simulink model "pBrake"  (R2024b)
settings: Solver=FixedStepDiscrete  StartTime=0.0  StopTime=1  FixedStep=0.001  RelTol=1e-3  EnableMultiTasking=on
undefined symbols (not defined in the file): pBrakeGain
settings Model: DataDictionary=Master_Dictionary.sldd  EnableAccessToBaseWorkspace=off  Creator=rubyg  LastModifiedBy=oxbro
settings SolverCC: AlgebraicLoopSolver=TrustRegion
settings DataIOCC: ReturnWorkspaceOutputs=off
settings OptimizationCC: DefaultParameterBehavior=Inlined  EnhancedBackFolding=on  PassReuseOutputArgsAs=Individual arguments  ZeroExternalMemoryAtStartup=off  ZeroInternalMemoryAtStartup=off  MaxStackSize=512  OptimizeBlockOrder=speed  DifferentSizesBufferReuse=on  OptimizationCustomize=off  EfficientTunableParamExpr=on
settings DebuggingCC: ParameterTunabilityLossMsg=error  UnconnectedInputMsg=warning  UnconnectedOutputMsg=warning  UnconnectedLineMsg=warning  ArithmeticOperatorsInVariantConditions=warning
settings HardwareCC: ProdBitPerPointer=32  ProdBitPerSizeT=32  ProdBitPerPtrDiffT=32  ProdLargestAtomicInteger=Long  ProdLargestAtomicFloat=Double  ProdWordSize=32  ProdLongLongMode=on  ProdHWDeviceType=ARM Compatible->ARM Cortex-M
settings ModelReferenceCC: EnableRefExpFcnMdlSchedulingChecks=on
settings SFSimCC: MATLABDynamicMemAlloc=off  CustomCodeUndefinedFunction=UseInterfaceOnly
settings RTWCC: Description=Embedded Coder  SystemTargetFile=ert.tlc  HardwareBoard=STM32H7xx Based (Single-core)  TemplateMakefile=ert_default_tmf  CustomHeaderCode="#include \"stm32h7xx_ll_tim.h\""  CustomInitializer=LL_TIM_EnableCounter(TIM2);  Toolchain=GNU Tools for ARM Embedded Processors  GPUComputeCapability=3.5
settings CodeAppCC: ForceParamTrailComments=on  IgnoreCustomStorageClasses=off  OperatorAnnotations=on  SimulinkDataObjDesc=on  SFDataObjDesc=on  InsertBlockDesc=on
settings ERTTargetCC: TargetLangStandard=C99 (ISO)  CodeReplacementLibrary=ARM Cortex-M  ExtModeTransport=3  ExtModeStaticAlloc=on  ExtModeStaticAllocSize=2048  ExtModeMexFile=ext_xcp  ExtModeIntrfLevel=Level2 - Open

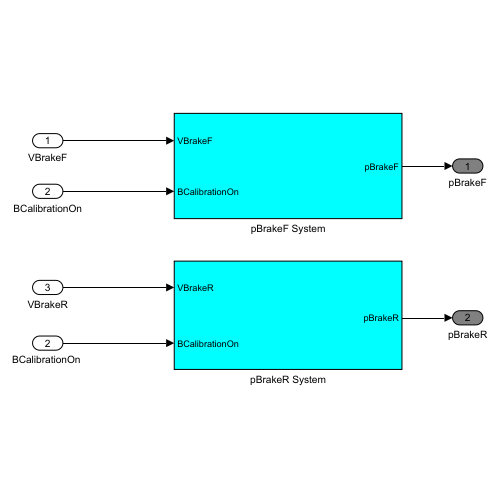
[thumbnail: Simulink's stored preview of the top-level diagram]
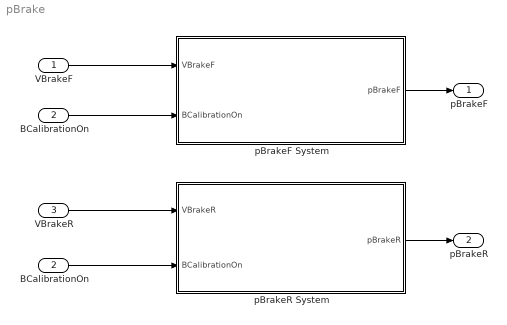
== system pBrake ==
  VBrakeF : Inport
  BCalibrationOn : Inport  Port=2  OutDataTypeStr=boolean
  VBrakeR : Inport  Port=3
  "BCalibrationOn " : InportShadow  Port=2  OutDataTypeStr=boolean
  pBrakeF System : Subsystem
  pBrakeR System : Subsystem
  pBrakeF : Outport  OutDataTypeStr=double  VectorParamsAs1DForOutWhenUnconnected=off
  pBrakeR : Outport  Port=2  OutDataTypeStr=double  VectorParamsAs1DForOutWhenUnconnected=off
  wires:
  BCalibrationOn/1 -> pBrakeF System/2(BCalibrationOn)
  VBrakeF/1 -> pBrakeF System/1(VBrakeF)
  "BCalibrationOn "/1 -> pBrakeR System/2(BCalibrationOn)
  VBrakeR/1 -> pBrakeR System/1(VBrakeR)
  pBrakeF System/1(pBrakeF) -> pBrakeF/1
  pBrakeR System/1(pBrakeR) -> pBrakeR/1

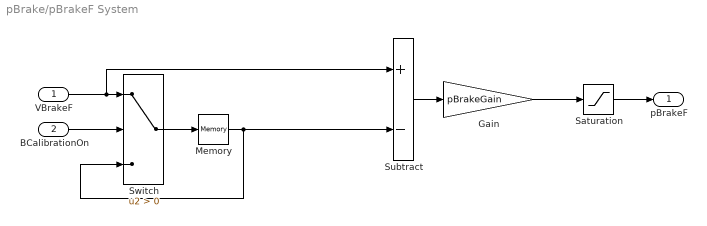
== system pBrake/pBrakeF System ==
  VBrakeF : Inport
  BCalibrationOn : Inport  Port=2  OutDataTypeStr=boolean
  Gain : Gain  Gain=pBrakeGain
  Memory : Memory  InitialCondition=500  InheritSampleTime=on
  Saturation : Saturate  UpperLimit=240  LowerLimit=-80
  Subtract : Sum  Inputs=+-
  Switch : Switch  Criteria=u2 > Threshold  SaturateOnIntegerOverflow=off  InputSameDT=off
  pBrakeF : Outport  VectorParamsAs1DForOutWhenUnconnected=off
  wires:
  VBrakeF/1 -> Subtract/1, Switch/1
  BCalibrationOn/1 -> Switch/2
  Switch/1 -> Memory/1
  Memory/1 -> Switch/3, Subtract/2
  Subtract/1 -> Gain/1
  Saturation/1 -> pBrakeF/1
  Gain/1 -> Saturation/1

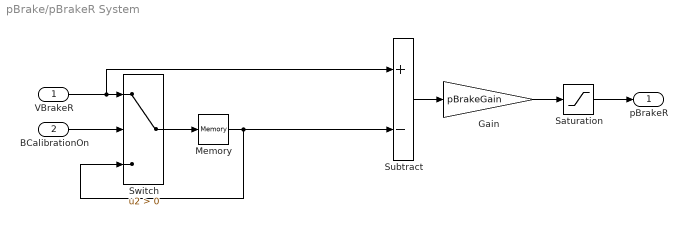
== system pBrake/pBrakeR System ==
  VBrakeR : Inport
  BCalibrationOn : Inport  Port=2  OutDataTypeStr=boolean
  Gain : Gain  Gain=pBrakeGain
  Memory : Memory  InitialCondition=500  InheritSampleTime=on
  Saturation : Saturate  UpperLimit=240  LowerLimit=-80
  Subtract : Sum  Inputs=+-
  Switch : Switch  Criteria=u2 > Threshold  SaturateOnIntegerOverflow=off  InputSameDT=off
  pBrakeR : Outport  VectorParamsAs1DForOutWhenUnconnected=off
  wires:
  Saturation/1 -> pBrakeR/1
  Subtract/1 -> Gain/1
  Memory/1 -> Switch/3, Subtract/2
  Switch/1 -> Memory/1
  BCalibrationOn/1 -> Switch/2
  VBrakeR/1 -> Switch/1, Subtract/1
  Gain/1 -> Saturation/1
